simulink model "gm_ddc_simulink_CRD_fixed"  (R2022b)
settings: Solver=FixedStepDiscrete  StartTime=0.0  StopTime=0.005  FixedStep=1/Fs  RelTol=1e-3
libraries: dsphdlsigops2 x2, hdlmdlgenlib x1
settings Model: FPTRunName=BaselineRun  Creator=caleb  LastModifiedBy=caleb
settings OptimizationCC: BlockReduction=off  ConditionallyExecuteInputs=off
settings DebuggingCC: SignalRangeChecking=warning  InheritedTsInSrcMsg=none  SingleTaskRateTransMsg=error

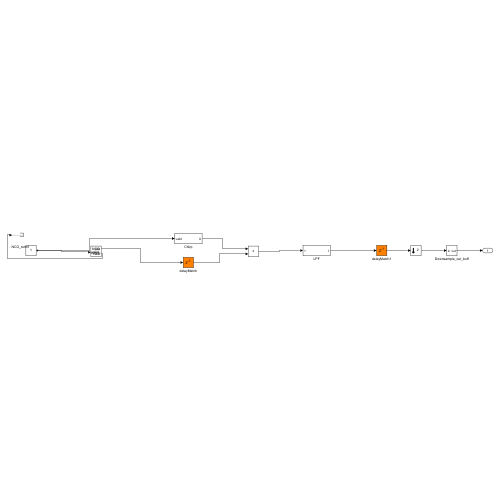
[thumbnail: Simulink's stored preview of the top-level diagram]
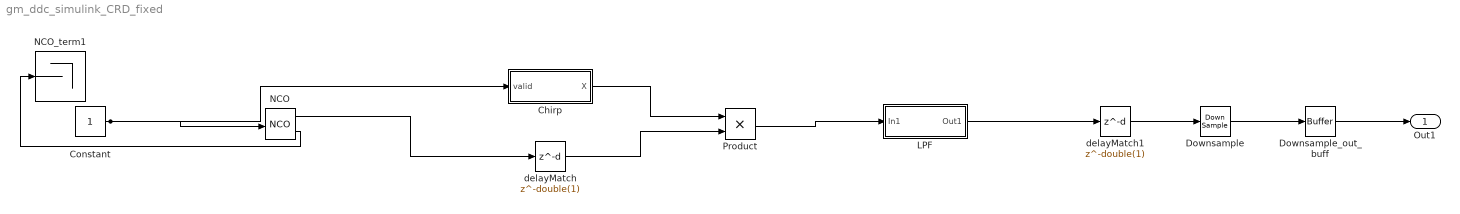
== system gm_ddc_simulink_CRD_fixed ==
  Chirp : Subsystem
  Constant : Constant  OutDataTypeStr=boolean  SampleTime=1.66666666666667e-08
  Downsample : DownSample  N=double(2)  phase=double(0)  RateOptions=Allow multirate processing  AllowArbitraryFixedInput=on
  Downsample_out_buff : hdlmdlgenlib/Buffer
  LPF : Subsystem
  NCO : dsphdlsigops2/NCO  PhaseIncrementSource=Property  PhaseIncrement=phIncr  PhaseOffsetSource=Property  PhaseOffset=phOff  DitherSource=Property  NumDitherBits=ditherBits  SamplesPerFrame=1  LUTCompress=off  ResetAction=off  Waveform=Cosine  PhasePort=off  SimulateUsing=Code generation  AccumulatorWL=N  PhaseQuantization=on  NumQuantizerAccumulatorBits=Q  OutputDataType=Binary point scaling  OutputWL=16  OutputFL=14
  NCO_term1 : Terminator
  Product : Product  Inputs=**  OutDataTypeStr=fixdt(1, 16, 14)  SampleTime=1.66666666666667e-08
  delayMatch : Delay  DelayLength=double(1)  InitialCondition=0  SampleTime=1.66666666666667e-08
  delayMatch1 : Delay  DelayLength=double(1)  InitialCondition=0  SampleTime=1.66666666666667e-08
  Out1 : Outport  SampleTime=3.33333333333333e-08  VectorParamsAs1DForOutWhenUnconnected=off
  wires:
  Chirp/1(X) -> Product/1
  Downsample_out_buff/1 -> Out1/1
  delayMatch1/1 -> Downsample/1
  delayMatch/1 -> Product/2
  NCO/2 -> NCO_term1/1
  Product/1 -> LPF/1(In1)
  Constant/1 -> Chirp/1(valid), NCO/1
  Downsample/1 -> Downsample_out_buff/1
  NCO/1 -> delayMatch/1
  LPF/1(Out1) -> delayMatch1/1

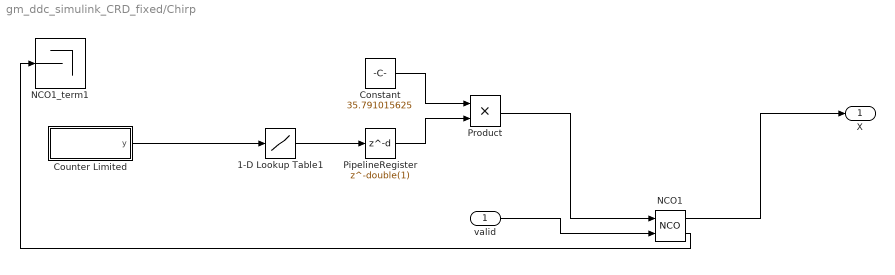
== system gm_ddc_simulink_CRD_fixed/Chirp ==
  valid : Inport  OutDataTypeStr=boolean  PortDimensions=1  SampleTime=1.66666666666667e-08
  1-D Lookup Table1 : Lookup_n-D  NumberOfTableDimensions=1  BreakpointsForDimension1="fi(\"numerictype\",numerictype(0,16,0),\"fimath\",fimath(\"RoundingMethod\", \"Nearest\",\"OverflowAction\", \"Saturate\",\"ProductMode\",\"FullPrecision\",\"SumMode\",\"FullPrecision\"),\"Value\",\"[0 1 2 3 4 5 6 7 8 9 10 11 12 13 14 15 16 17 18 19 20 21 22 23 24 25 26 27 28 29 30 31 32 33 34 35 36 37 38 39 40 41 42 43 44 45 46 47 48 49 50 51 52 53 54 55 56 57 58 59 60 61 62 63 64 65 66 67 68 69 70 71 72 73 74 75 76 77 78 79 80 81 82 83 84 85 86 87 88 89 90 91 92 93 94 95 96 97 98 99 100 101 102 103 104 105 106 107 108 109 110 111 112 113 114 115 116 117 118 119 120 121 122 123 124 125 126 127 128 129 130 131 132 133 134 135 136 137 138 139 140 141 142 143 144 145 146 147 148 149 150 151 152 153 154 155 156 157 158 159 160 161 162 163 164 165 166 167 168 169 170 171 172 173 174 175 176 177 178 179 180 181 182 183 184 185 186 187 188 189 190 191 192 193 194 195 196 197 198 199 200 201 202 203 204 205 206 207 208 209 210 211 212 213 214 215 216 217 218 219 220 221 222 223 224 225 226 227 228 229 230 231 232 233 234 235 236 237 238 239 240 241 242 243 244 245 246 247 248 249 250 251 252 253 254 255 256 257 258 259 260 261 262 263 264 265 266 267 268 269 270 271 272 273 274 275 276 277 278 279 280 281 282 283 284 285 286 287 288 289 290 291 292 293 294 295 296 297 298 299 300 301 302 303 304 305 306 307 308 309 310 311 312 313 314 315 316 317 318 319 320 321 322 323 324 325 326 327 328 329 330 331 332 333 334 335 336 337 338 339 340 341 342 343 344 345 346 347 348 349 350 351 352 353 354 355 356 357 358 359 360 361 362 363 364 365 366 367 368 369 370 371 372 373 374 375 376 377 378 379 380 381 382 383 384 385 386 387 388 389 390 391 392 393 394 395 396 397 398 399 400 401 402 403 404 405 406 407 408 409 410 411 412 413 414 415 416 417 418 419 420 421 422 423 424 425 426 427 428 429 430 431 432 433 434 435 436 437 438 439 440 441 442 443 444 445 446 447 448 449 450 451 452 453 454 455 456 457 458 459 460 461 462 463 464 465 466 467 468 469 470 471 472 473 474 475 476 477 478 479 480 481 482 483 484 485 486 487 488 489 490 491 492 493 494 495 496 497 498 499 500 501 502 503 504 505 506 507 508 509 510 511 512 513 514 515 516 517 518 519 520 521 522 523 524 525 526 527 528 529 530 531 532 533 534 535 536 537 538 539 540 541 542 543 544 545 546 547 548 549 550 551 552 553 554 555 556 557 558 559 560 561 562 563 564 565 566 567 568 569 570 571 572 573 574 575 576 577 578 579 580 581 582 583 584 585 586 587 588 589 590 591 592 593 594 595 596 597 598 599 600 601 602 603 604 605 606 607 608 609 610 611 612 613 614 615 616 617 618 619 620 621 622 623 624 625 626 627 628 629 630 631 632 633 634 635 636 637 638 639 640 641 642 643 644 645 646 647 648 649 650 651 652 653 654 655 656 657 658 659 660 661 662 663 664 665 666 667 668 669 670 671 672 673 674 675 676 677 678 679 680 681 682 683 684 685 686 687 688 689 690 691 692 693 694 695 696 697 698 699 700 701 702 703 704 705 706 707 708 709 710 711 712 713 714 715 716 717 718 719 720 721 722 723 724 725 726 727 728 729 730 731 732 733 734 735 736 737 738 739 740 741 742 743 744 745 746 747 748 749 750 751 752 753 754 755 756 757 758 759 760 761 762 763 764 765 766 767 768 769 770 771 772 773 774 775 776 777 778 779 780 781 782 783 784 785 786 787 788 789 790 791 792 793 794 795 796 797 798 799 800 801 802 803 804 805 806 807 808 809 810 811 812 813 814 815 816 817 818 819 820 821 822 823 824 825 826 827 828 829 830 831 832 833 834 835 836 837 838 839 840 841 842 843 844 845 846 847 848 849 850 851 852 853 854 855 856 857 858 859 860 861 862 863 864 865 866 867 868 869 870 871 872 873 874 875 876 877 878 879 880 881 882 883 884 885 886 887 888 889 890 891 892 893 894 895 896 897 898 899 900 901 902 903 904 905 906 907 908 909 910 911 912 913 914 915 916 917 918 919 920 921 922 923 924 925 926 927 928 929 930 931 932 933 934 935 936 937 938 939 940 941 942 943 944 945 946 947 948 949 950 951 952 953 954 955 956 957 958 959 960 961 962 963 964 965 966 967 968 969 970 971 972 973 974 975 976 977 978 979 980 981 982 983 984 985 986 987 988 989 990 991 992 993 994 995 996 997 998 999 1000 1001 1002 1003 1004 1005 1006 1007 1008 1009 1010 1011 1012 1013 1014 1015 1016 1017 1018 1019 1020 ...(+900 chars)]\")"  Table="reshape(fi(\"numerictype\",numerictype(0,32,0),\"fimath\",fimath(\"RoundingMethod\", \"Floor\",\"OverflowAction\", \"Wrap\",\"ProductMode\",\"FullPrecision\",\"SumMode\",\"FullPrecision\"),\"Value\",\"[10000000;10008333;10016667;10025000;10033333;10041667;10050000;10058333;10066667;10075000;10083333;10091667;10100000;10108333;10116667;10125000;10133333;10141667;10150000;10158333;10166667;10175000;10183333;10191667;10200000;10208333;10216667;10225000;10233333;10241667;10250000;10258333;10266667;10275000;10283333;10291667;10300000;10308333;10316667;10325000;10333333;10341667;10350000;10358333;10366667;10375000;10383333;10391667;10400000;10408333;10416667;10425000;10433333;10441667;10450000;10458333;10466667;10475000;10483333;10491667;10500000;10508333;10516667;10525000;10533333;10541667;10550000;10558333;10566667;10575000;10583333;10591667;10600000;10608333;10616667;10625000;10633333;10641667;10650000;10658333;10666667;10675000;10683333;10691667;10700000;10708333;10716667;10725000;10733333;10741667;10750000;10758333;10766667;10775000;10783333;10791667;10800000;10808333;10816667;10825000;10833333;10841667;10850000;10858333;10866667;10875000;10883333;10891667;10900000;10908333;10916667;10925000;10933333;10941667;10950000;10958333;10966667;10975000;10983333;10991667;11000000;11008333;11016667;11025000;11033333;11041667;11050000;11058333;11066667;11075000;11083333;11091667;11100000;11108333;11116667;11125000;11133333;11141667;11150000;11158333;11166667;11175000;11183333;11191667;11200000;11208333;11216667;11225000;11233333;11241667;11250000;11258333;11266667;11275000;11283333;11291667;11300000;11308333;11316667;11325000;11333333;11341667;11350000;11358333;11366667;11375000;11383333;11391667;11400000;11408333;11416667;11425000;11433333;11441667;11450000;11458333;11466667;11475000;11483333;11491667;11500000;11508333;11516667;11525000;11533333;11541667;11550000;11558333;11566667;11575000;11583333;11591667;11600000;11608333;11616667;11625000;11633333;11641667;11650000;11658333;11666667;11675000;11683333;11691667;11700000;11708333;11716667;11725000;11733333;11741667;11750000;11758333;11766667;11775000;11783333;11791667;11800000;11808333;11816667;11825000;11833333;11841667;11850000;11858333;11866667;11875000;11883333;11891667;11900000;11908333;11916667;11925000;11933333;11941667;11950000;11958333;11966667;11975000;11983333;11991667;12000000;12008333;12016667;12025000;12033333;12041667;12050000;12058333;12066667;12075000;12083333;12091667;12100000;12108333;12116667;12125000;12133333;12141667;12150000;12158333;12166667;12175000;12183333;12191667;12200000;12208333;12216667;12225000;12233333;12241667;12250000;12258333;12266667;12275000;12283333;12291667;12300000;12308333;12316667;12325000;12333333;12341667;12350000;12358333;12366667;12375000;12383333;12391667;12400000;12408333;12416667;12425000;12433333;12441667;12450000;12458333;12466667;12475000;12483333;12491667;12500000;12508333;12516667;12525000;12533333;12541667;12550000;12558333;12566667;12575000;12583333;12591667;12600000;12608333;12616667;12625000;12633333;12641667;12650000;12658333;12666667;12675000;12683333;12691667;12700000;12708333;12716667;12725000;12733333;12741667;12750000;12758333;12766667;12775000;12783333;12791667;12800000;12808333;12816667;12825000;12833333;12841667;12850000;12858333;12866667;12875000;12883333;12891667;12900000;12908333;12916667;12925000;12933333;12941667;12950000;12958333;12966667;12975000;12983333;12991667;13000000;13008333;13016667;13025000;13033333;13041667;13050000;13058333;13066667;13075000;13083333;13091667;13100000;13108333;13116667;13125000;13133333;13141667;13150000;13158333;13166667;13175000;13183333;13191667;13200000;13208333;13216667;13225000;13233333;13241667;13250000;13258333;13266667;13275000;13283333;13291667;13300000;13308333;13316667;13325000;13333333;13341667;13350000;13358333;13366667;13375000;13383333;13391667;13400000;13408333;13416667;13425000;13433333;13441667;13450000;13458333;13466667;13475000;13483333;13491667;13500000;13508333;13516667;13525000;13533333;13541667;13550000;13558333;13566667;13575000;13583333;13591667;13600000;13608333;13616667;13625000;13633333;13641667;13650000;13658333;13666667;13675000;13683333;13691667 ...(+6813 chars)]\"), [1  1201])"  InterpMethod=Flat  ExtrapMethod=Clip  DiagnosticForOutOfRangeInput=Error  SampleTime=1.66666666666667e-08  OutDataTypeStr=uint32  RndMeth=Simplest
  Constant : Constant  Value=35.791015625  OutDataTypeStr=fixdt(0, 16, 10)  SampleTime=1.66666666666667e-08
  Counter Limited : Subsystem  mask(Counter Limited){uplimit=double(3.3333333333333334e-13), tsamp=double(1.6666666666666667e-08)}
      mask prompts: uplimit "Simulink:masks:UpperLimit_MP"; tsamp "Simulink:masks:SampleTime_MP"
      mask help: Simulink:masks:CounterLimited_MD
      mask init:
      | nbits = double(8);
      | tsamp = double(1.6666666666666667e-08);
      | uplimit = double(3.3333333333333334e-13);
  NCO1 : dsphdlsigops2/NCO  PhaseIncrementSource=Input port  PhaseIncrement=phIncr  PhaseOffsetSource=Property  PhaseOffset=phOff  DitherSource=Property  NumDitherBits=ditherBits  SamplesPerFrame=1  LUTCompress=off  ResetAction=off  Waveform=Cosine  PhasePort=off  SimulateUsing=Code generation  AccumulatorWL=N  PhaseQuantization=on  NumQuantizerAccumulatorBits=Q  OutputDataType=Binary point scaling  OutputWL=16  OutputFL=14
  NCO1_term1 : Terminator
  PipelineRegister : Delay  DelayLength=double(1)  InitialCondition=0  SampleTime=1.66666666666667e-08
  Product : Product  Inputs=**  OutDataTypeStr=uint32  SampleTime=1.66666666666667e-08
  X : Outport  SampleTime=1.66666666666667e-08
  wires:
  PipelineRegister/1 -> Product/2
  Constant/1 -> Product/1
  Counter Limited/1(y) -> 1-D Lookup Table1/1
  NCO1/1 -> X/1
  NCO1/2 -> NCO1_term1/1
  Product/1 -> NCO1/1
  valid/1 -> NCO1/2
  1-D Lookup Table1/1 -> PipelineRegister/1

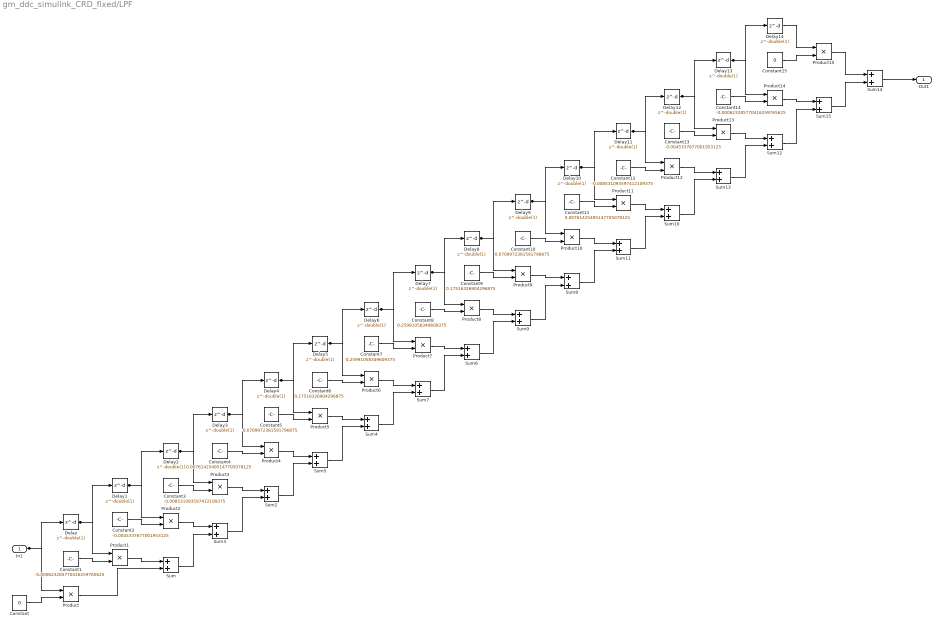
== system gm_ddc_simulink_CRD_fixed/LPF ==
  In1 : Inport  OutDataTypeStr=fixdt(1, 16, 14)  PortDimensions=1  SampleTime=1.66666666666667e-08
  Constant : Constant  Value=0  OutDataTypeStr=fixdt(1, 16, 4)  SampleTime=1.66666666666667e-08
  Constant1 : Constant  Value=-0.000623285770416259765625  OutDataTypeStr=fixdt(1, 16, 25)  SampleTime=1.66666666666667e-08
  Constant10 : Constant  Value=0.0709972381591796875  OutDataTypeStr=fixdt(0, 16, 19)  SampleTime=1.66666666666667e-08
  Constant11 : Constant  Value=0.00761425495147705078125  OutDataTypeStr=fixdt(0, 16, 23)  SampleTime=1.66666666666667e-08
  Constant12 : Constant  Value=-0.008531093597412109375  OutDataTypeStr=fixdt(1, 16, 21)  SampleTime=1.66666666666667e-08
  Constant13 : Constant  Value=-0.0045337677001953125  OutDataTypeStr=fixdt(1, 16, 22)  SampleTime=1.66666666666667e-08
  Constant14 : Constant  Value=-0.000623285770416259765625  OutDataTypeStr=fixdt(1, 16, 25)  SampleTime=1.66666666666667e-08
  Constant15 : Constant  Value=0  OutDataTypeStr=fixdt(1, 16, 4)  SampleTime=1.66666666666667e-08
  Constant2 : Constant  Value=-0.0045337677001953125  OutDataTypeStr=fixdt(1, 16, 22)  SampleTime=1.66666666666667e-08
  Constant3 : Constant  Value=-0.008531093597412109375  OutDataTypeStr=fixdt(1, 16, 21)  SampleTime=1.66666666666667e-08
  Constant4 : Constant  Value=0.00761425495147705078125  OutDataTypeStr=fixdt(0, 16, 23)  SampleTime=1.66666666666667e-08
  Constant5 : Constant  Value=0.0709972381591796875  OutDataTypeStr=fixdt(0, 16, 19)  SampleTime=1.66666666666667e-08
  Constant6 : Constant  Value=0.17516326904296875  OutDataTypeStr=fixdt(0, 16, 18)  SampleTime=1.66666666666667e-08
  Constant7 : Constant  Value=0.25991058349609375  OutDataTypeStr=fixdt(0, 16, 17)  SampleTime=1.66666666666667e-08
  Constant8 : Constant  Value=0.25991058349609375  OutDataTypeStr=fixdt(0, 16, 17)  SampleTime=1.66666666666667e-08
  Constant9 : Constant  Value=0.17516326904296875  OutDataTypeStr=fixdt(0, 16, 18)  SampleTime=1.66666666666667e-08
  Delay{,1..14} (15 alike) : Delay  DelayLength=double(1)  InitialCondition=0  SampleTime=1.66666666666667e-08
  Product : Product  Inputs=**  OutDataTypeStr=fixdt(1, 16, 4)  SampleTime=1.66666666666667e-08
  Product1 : Product  Inputs=**  OutDataTypeStr=fixdt(1, 16, 25)  SampleTime=1.66666666666667e-08
  Product10 : Product  Inputs=**  OutDataTypeStr=fixdt(1, 16, 18)  SampleTime=1.66666666666667e-08
  Product{2,4,11,13} (4 alike) : Product  Inputs=**  OutDataTypeStr=fixdt(1, 16, 22)  SampleTime=1.66666666666667e-08
  Product12 : Product  Inputs=**  OutDataTypeStr=fixdt(1, 16, 21)  SampleTime=1.66666666666667e-08
  Product14 : Product  Inputs=**  OutDataTypeStr=fixdt(1, 16, 25)  SampleTime=1.66666666666667e-08
  Product15 : Product  Inputs=**  OutDataTypeStr=fixdt(1, 16, 4)  SampleTime=1.66666666666667e-08
  Product3 : Product  Inputs=**  OutDataTypeStr=fixdt(1, 16, 21)  SampleTime=1.66666666666667e-08
  Product5 : Product  Inputs=**  OutDataTypeStr=fixdt(1, 16, 18)  SampleTime=1.66666666666667e-08
  Product6 : Product  Inputs=**  OutDataTypeStr=fixdt(1, 16, 17)  SampleTime=1.66666666666667e-08
  Product7 : Product  Inputs=**  OutDataTypeStr=fixdt(1, 16, 16)  SampleTime=1.66666666666667e-08
  Product8 : Product  Inputs=**  OutDataTypeStr=fixdt(1, 16, 16)  SampleTime=1.66666666666667e-08
  Product9 : Product  Inputs=**  OutDataTypeStr=fixdt(1, 16, 17)  SampleTime=1.66666666666667e-08
  Sum : Sum  AccumDataTypeStr=fixdt(1, 32, 25)  OutDataTypeStr=fixdt(1, 16, 25)  SampleTime=1.66666666666667e-08
  Sum10 : Sum  AccumDataTypeStr=fixdt(1, 32, 22)  OutDataTypeStr=fixdt(1, 16, 16)  SampleTime=1.66666666666667e-08
  Sum11 : Sum  AccumDataTypeStr=fixdt(1, 32, 18)  OutDataTypeStr=fixdt(1, 16, 16)  SampleTime=1.66666666666667e-08
  Sum12 : Sum  AccumDataTypeStr=fixdt(1, 32, 22)  OutDataTypeStr=fixdt(1, 16, 16)  SampleTime=1.66666666666667e-08
  Sum13 : Sum  AccumDataTypeStr=fixdt(1, 32, 21)  OutDataTypeStr=fixdt(1, 16, 16)  SampleTime=1.66666666666667e-08
  Sum14 : Sum  AccumDataTypeStr=fixdt(1, 32, 16)  OutDataTypeStr=fixdt(1, 16, 16)  SampleTime=1.66666666666667e-08
  Sum15 : Sum  AccumDataTypeStr=fixdt(1, 32, 25)  OutDataTypeStr=fixdt(1, 16, 16)  SampleTime=1.66666666666667e-08
  Sum2 : Sum  AccumDataTypeStr=fixdt(1, 32, 22)  OutDataTypeStr=fixdt(1, 16, 21)  SampleTime=1.66666666666667e-08
  Sum3 : Sum  AccumDataTypeStr=fixdt(1, 32, 25)  OutDataTypeStr=fixdt(1, 16, 22)  SampleTime=1.66666666666667e-08
  Sum4 : Sum  AccumDataTypeStr=fixdt(1, 32, 21)  OutDataTypeStr=fixdt(1, 16, 18)  SampleTime=1.66666666666667e-08
  Sum5 : Sum  AccumDataTypeStr=fixdt(1, 32, 22)  OutDataTypeStr=fixdt(1, 16, 21)  SampleTime=1.66666666666667e-08
  Sum6 : Sum  AccumDataTypeStr=fixdt(1, 32, 17)  OutDataTypeStr=fixdt(1, 16, 16)  SampleTime=1.66666666666667e-08
  Sum7 : Sum  AccumDataTypeStr=fixdt(1, 32, 18)  OutDataTypeStr=fixdt(1, 16, 17)  SampleTime=1.66666666666667e-08
  Sum8 : Sum  AccumDataTypeStr=fixdt(1, 32, 17)  OutDataTypeStr=fixdt(1, 16, 16)  SampleTime=1.66666666666667e-08
  Sum9 : Sum  AccumDataTypeStr=fixdt(1, 32, 16)  OutDataTypeStr=fixdt(1, 16, 16)  SampleTime=1.66666666666667e-08
  Out1 : Outport  SampleTime=1.66666666666667e-08
  wires:
  Constant/1 -> Product/2
  Constant1/1 -> Product1/2
  Constant10/1 -> Product10/2
  Constant11/1 -> Product11/2
  Constant12/1 -> Product12/2
  Constant13/1 -> Product13/2
  Constant14/1 -> Product14/2
  Constant15/1 -> Product15/2
  Constant2/1 -> Product2/2
  Constant3/1 -> Product3/2
  Constant4/1 -> Product4/2
  Constant5/1 -> Product5/2
  Constant6/1 -> Product6/2
  Constant7/1 -> Product7/2
  Constant8/1 -> Product8/2
  Constant9/1 -> Product9/2
  Delay/1 -> Product1/1, Delay1/1
  Delay1/1 -> Product2/1, Delay2/1
  Delay10/1 -> Product11/1, Delay11/1
  Delay11/1 -> Product12/1, Delay12/1
  Delay12/1 -> Product13/1, Delay13/1
  Delay13/1 -> Product14/1, Delay14/1
  Delay14/1 -> Product15/1
  Delay2/1 -> Product3/1, Delay3/1
  Delay3/1 -> Product4/1, Delay4/1
  Delay4/1 -> Product5/1, Delay5/1
  Delay5/1 -> Product6/1, Delay6/1
  Delay6/1 -> Product7/1, Delay7/1
  Delay7/1 -> Product8/1, Delay8/1
  Delay8/1 -> Product9/1, Delay9/1
  Delay9/1 -> Product10/1, Delay10/1
  Product/1 -> Sum/2
  Product1/1 -> Sum/1
  Product10/1 -> Sum11/1
  Product11/1 -> Sum10/1
  Product12/1 -> Sum13/1
  Product13/1 -> Sum12/1
  Product14/1 -> Sum15/1
  Product15/1 -> Sum14/1
  Product2/1 -> Sum3/1
  Product3/1 -> Sum2/1
  Product4/1 -> Sum5/1
  Product5/1 -> Sum4/1
  Product6/1 -> Sum7/1
  Product7/1 -> Sum6/1
  Product8/1 -> Sum9/1
  Product9/1 -> Sum8/1
  Sum/1 -> Sum3/2
  Sum10/1 -> Sum13/2
  Sum11/1 -> Sum10/2
  Sum12/1 -> Sum15/2
  Sum13/1 -> Sum12/2
  Sum14/1 -> Out1/1
  Sum15/1 -> Sum14/2
  Sum2/1 -> Sum5/2
  Sum3/1 -> Sum2/2
  Sum4/1 -> Sum7/2
  Sum5/1 -> Sum4/2
  Sum6/1 -> Sum9/2
  Sum7/1 -> Sum6/2
  Sum8/1 -> Sum11/2
  Sum9/1 -> Sum8/2
  In1/1 -> Product/1, Delay/1

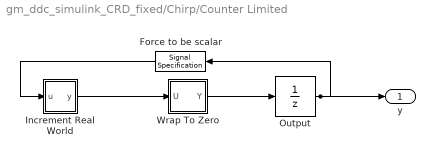
== system gm_ddc_simulink_CRD_fixed/Chirp/Counter Limited ==
  Force to be scalar : SignalSpecification  DisableCoverage=on  Dimensions=1
  Increment Real World : Subsystem  mask(Real World Value Increment){}
      mask help: Simulink:masks:RealWorldValueIncrement_MD
      mask Display: disp('V++')
  Output : UnitDelay  InitialCondition=0.0  SampleTime=tsamp  HasFrameUpgradeWarning=on
  Wrap To Zero : Subsystem  mask(Wrap To Zero){Threshold=double(3.3333333333333334e-13)}
      mask prompts: Threshold "Simulink:masks:Threshold_MP"
      mask help: Simulink:masks:WrapToZero_MD
  y : Outport  SampleTime=1.66666666666667e-08
  wires:
  Output/1 -> y/1, Force to be scalar/1
  Force to be scalar/1 -> Increment Real World/1(u)
  Increment Real World/1(y) -> Wrap To Zero/1(U)
  Wrap To Zero/1(Y) -> Output/1

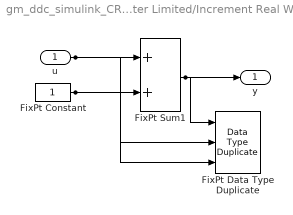
== system gm_ddc_simulink_CRD_fixed/Chirp/Counter Limited/Increment Real World ==
  u : Inport  OutDataTypeStr=uint8  SampleTime=1.66666666666667e-08
  FixPt Constant : Constant  DisableCoverage=on  OutDataTypeStr=Inherit: Inherit via back propagation  SampleTime=-1
  FixPt Data Type Duplicate : DataTypeDuplicate  DisableCoverage=on  NumInputPorts=3
  FixPt Sum1 : Sum  InputSameDT=on  OutDataTypeStr=Inherit: Inherit via back propagation  LockScale=on
  y : Outport  SampleTime=1.66666666666667e-08
  wires:
  FixPt Constant/1 -> FixPt Sum1/2, FixPt Data Type Duplicate/3
  FixPt Sum1/1 -> FixPt Data Type Duplicate/1, y/1
  u/1 -> FixPt Sum1/1, FixPt Data Type Duplicate/2

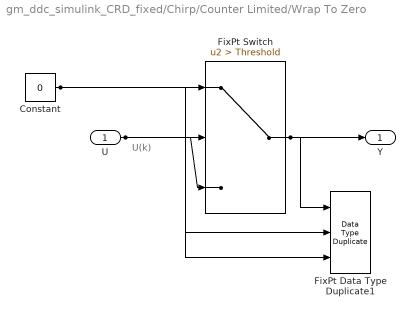
== system gm_ddc_simulink_CRD_fixed/Chirp/Counter Limited/Wrap To Zero ==
  note: U(k)
  U : Inport  OutDataTypeStr=uint8  SampleTime=1.66666666666667e-08
  Constant : Constant  DisableCoverage=on  Value=0  OutDataTypeStr=Inherit: Inherit via back propagation  SampleTime=-1
  FixPt Data Type Duplicate1 : DataTypeDuplicate  DisableCoverage=on  NumInputPorts=3
  FixPt Switch : Switch  Criteria=u2 > Threshold  Threshold=Threshold  OutDataTypeStr=Inherit: Inherit via back propagation  ZeroCross=off  SaturateOnIntegerOverflow=off  InputSameDT=off
  Y : Outport  SampleTime=1.66666666666667e-08
  wires:
  Constant/1 -> FixPt Switch/1, FixPt Data Type Duplicate1/3
  FixPt Switch/1 -> FixPt Data Type Duplicate1/1, Y/1
  U/1 -> FixPt Switch/3, FixPt Switch/2, FixPt Data Type Duplicate1/2
